simulink model "PMSM_simscape_Model_vs_eq_dq_model"  (R2020b)
settings: Solver=ode23tb  StartTime=0.0  StopTime=0.1  RelTol=1e-4
InitFcn:
  | Ts_sim=20e-06;
  | p=2;
  | phimg=0.125;
  | Zp=2;
  | Rs=2.98;
  | Ld=7e-3;
  | Lq=7e-3;
  | Phimg=0.125;
  | Jm=0.47e-4;
  | Bv=11e-5;
  | TL=0;
  | Vdc=100;
libraries: powerlib x8, powerlib_meascontrol x1
settings Model: ExtModeTrigMode=oneshot  ExtModeArmWhenConnect=off  ExtModeAutoUpdateStatusClock=off  Creator=MathWorks  LastModifiedBy=Karim
settings DataIOCC: ExternalInput=[]  SaveFormat=Array  SignalLoggingSaveFormat=ModelDataLogs  SaveOutput=off  SaveTime=off  ReturnWorkspaceOutputs=off  SignalLoggingName=sigsOut
settings OptimizationCC: BlockReduction=off  BooleanDataType=off  ExpressionDepthLimit=2147483647  InitFltsAndDblsToZero=on  EfficientMapNaN2IntZero=off  LifeSpan=inf
settings DebuggingCC: UnderspecifiedInitializationDetection=Classic  MergeDetectMultiDrivingBlocksExec=none  CheckExecutionContextPreStartOutputMsg=on  CheckExecutionContextRuntimeOutputMsg=on  SignalResolutionControl=TryResolveAllWithWarning  MultiTaskDSMMsg=warning  MultiTaskCondExecSysMsg=none  SigSpecEnsureSampleTimeMsg=none  FcnCallInpInsideContextMsg=warning  StateNameClashWarn=warning  SFUnexpectedBacktrackingDiag=warning  SFNoUnconditionalDefaultTransitionDiag=warning  SFExecutionAtInitializationDiag=none  ArithmeticOperatorsInVariantConditions=warning
settings HardwareCC: ProdBitPerPointer=32  ProdBitPerSizeT=32  ProdBitPerPtrDiffT=32  ProdLargestAtomicFloat=None  ProdIntDivRoundTo=Undefined  ProdEndianess=Unspecified  ProdWordSize=32  ProdHWDeviceType=32-bit Generic  TargetUnknown=on
settings ModelReferenceCC: PropagateSignalLabelsOutOfModel=off
settings SFSimCC: SimUseLocalCustomCode=off  CustomCodeUndefinedFunction=UseInterfaceOnly
settings RTWCC: RTWUseLocalCustomCode=off
settings CodeAppCC: StateflowObjectComments=on
settings GRTTargetCC: TargetLangStandard=C89/C90 (ANSI)  CombineOutputUpdateFcns=off  GRTInterface=on
settings ConfigComp: CovMetricSettings=dw  CovSaveCumulativeToWorkspaceVar=on  CovSaveSingleToWorkspaceVar=on  CovExternalEMLEnable=off  CovSFcnEnable=off
settings SimscapeCC: SimscapeNormalizeSystem=off  SimscapeNominalValues={1, 'bar'; 1, 'cm^3/s'; 1, 'bar*kg/s'; 1, 'kJ/kg'; 1, 'kW'; }

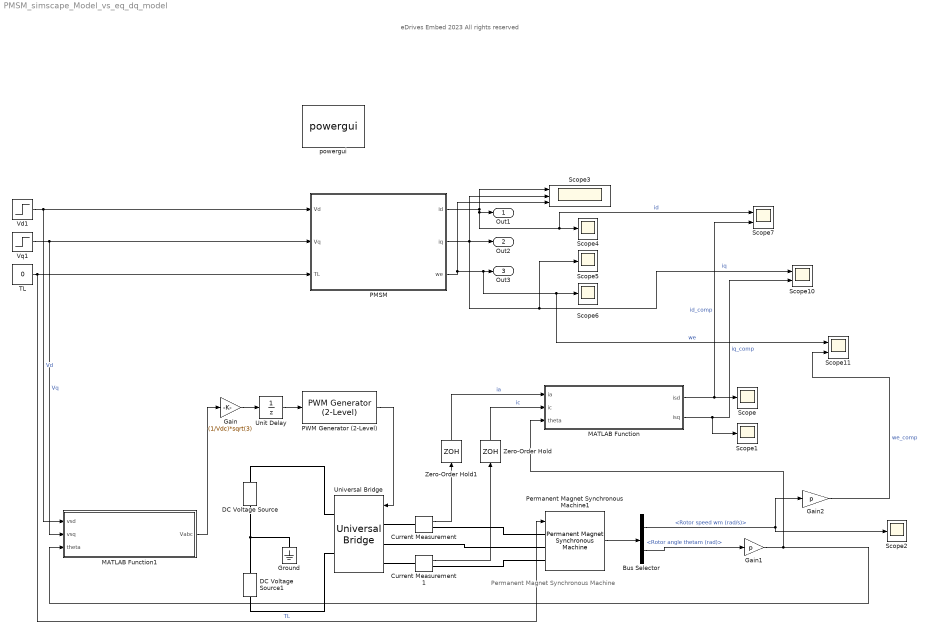
== system PMSM_simscape_Model_vs_eq_dq_model ==
  note: eDrives Embed
      | 2023 All rights reserved
  note: Permanent Magnet Synchronous Machine
  Bus Selector : BusSelector  OutputSignals=Rotor speed wm (rad/s),Rotor angle thetam (rad)
  Current Measurement : powerlib/Measurements/Current Measurement  PhasorSimulation=off  OutputType=Complex  PSBequivalent=0
  Current Measurement1 : powerlib/Measurements/Current Measurement  PhasorSimulation=off  OutputType=Complex  PSBequivalent=0
  DC Voltage Source : powerlib/Electrical Sources/DC Voltage Source  Amplitude=Vdc/2  Measurements=None
  DC Voltage Source1 : powerlib/Electrical Sources/DC Voltage Source  Amplitude=Vdc/2  Measurements=None
  Gain : Gain  Gain=(1/Vdc)*sqrt(3)
  Gain1 : Gain  Gain=p
  Gain2 : Gain  Gain=p
  Ground : powerlib/Elements/Ground  LConnTagsString=a
  MATLAB Function : MATLAB Function  TreatAsAtomicUnit=on
  MATLAB Function1 : MATLAB Function  TreatAsAtomicUnit=on
  PMSM : Subsystem
      mask Display: image('pmsm.png'); % Use "Edit Image" on toolstrip to change.
  PWM Generator (2-Level) : powerlib_meascontrol/Pulse & Signal Generators/PWM Generator (2-Level)  ModulatorType=Three-phase bridge (6 pulses)  ModulatorMode=Unsynchronized  Fc=2e3  Pc=90  nF=27  MinMax="[ -1  1 ]"  SamplingTechnique=Natural  ModulatingSignals=off  m=0.8  Freq=60  Phase=0  Ts=Ts_sim  ShowCarrierOutport=off
  Permanent Magnet Synchronous Machine1 : powerlib/Machines/Permanent Magnet Synchronous Machine  NbPhases=3  FluxDistribution=Sinusoidal  RotorType=Round  MechanicalLoad=Torque Tm  PresetModel=No  ShowDetailedParameters=on  MeasurementBus=off  Resistance=Rs  Inductance=8.5e-3  dqInductances=[8.5e-3,8.5e-3]  La=Ld  MachineConstant=Flux linkage established by magnets (V.s)  Flux=Phimg  VoltageCst=45.345  TorqueCst=0.375  Flat=120  Mechanical=[Jm, Bv p]  PolePairs=4  InitialConditions=[0,0, 0,0]  InitialConditions5ph=[0 0 0 0 0 0]  RefAngle=Aligned with phase A axis (original Park)  IterativeDiscreteModel=Trapezoidal non iterative  TsBlock=-1  TsPowergui=0
  Scope{,1..2,4..6} (6 alike) : Scope
  Scope10 : Scope  NumInputPorts=2
  Scope11 : Scope  NumInputPorts=2
  Scope3 : Scope  NumInputPorts=3
  Scope7 : Scope  NumInputPorts=2
  TL : Constant  Value=0
  Unit Delay : UnitDelay  SampleTime=-1  HasFrameUpgradeWarning=on
  Universal Bridge : powerlib/Power Electronics/Universal Bridge  Arms=3  SnubberResistance=1e5  SnubberCapacitance=inf  Device=IGBT / Diodes  Ron=1e-3  Lon=0  ForwardVoltages="[  0  0  ]"  ForwardVoltage=0  GTOparameters=[ 10e-6 , 20e-6 ]  IGBTparameters=[ 1e-6 , 2e-6 ]  Measurements=None  Measurements_2=None  converterType=Rectifier
  Vd1 : Step  Time=0.001  After=5  SampleTime=0
  Vq1 : Step  Time=0.001  After=20  SampleTime=0
  Zero-Order Hold : ZeroOrderHold  SampleTime=100e-6
  Zero-Order Hold1 : ZeroOrderHold  SampleTime=100e-6
  powergui : powerlib/powergui  Priority=1  SimulationMode=Discrete  SampleTime=Ts_sim  frequency=60  Iterations=50  frequencyindice=0  Pbase=100e6  ErrMax=1e-4  UnitsV=kV  UnitsW=MW  buscounter=0  FunctionMessages=off  echomessages=off  EnableUseOfTLC=off  CurrentSourceSwitches=off  DisableSnubberDevices=off  DisableRonSwitches=off  DisableVfSwitches=off  DisplayEquations=off  AutomaticDiscreteSolvers=off  SolverType=Tustin/Backward Euler (TBE)  Interpol=off  ExternalGateDelay=off  methode=off  Ts=100  x0status=blocks  SPID=on  SwTol=0  HookPort=off  NonlinearTolerance=1e-4  nMaxIteration=100  ContinueOnMaxIteration=off  RestoreLinks=warning  ResistiveCurrentMeasurement=off  Frange=[0:2:500]  Ylog=off  Xlog=on  ShowGrid=off  save=off  variable=ZData  structure=0  ZoomFFT=off  StartTime=0.0  cycles=1  DisplayStyle=1  fundamental=60  FreqAxis=off  MaxFrequency=1000  frequencyindicesteady=1  RmsSteady=1  display=off
  Out1 : Outport
  Out2 : Outport  Port=2
  Out3 : Outport  Port=3
  wires:
  Bus Selector/1 -> Gain2/1, Scope2/1  "<Rotor speed wm (rad/s)>"
  Unit Delay/1 -> PWM Generator (2-Level)/1
  Gain1/1 -> MATLAB Function1/3(theta), MATLAB Function/3(theta)
  MATLAB Function/2(isq) -> Scope10/2, Scope1/1  "iq_comp"
  MATLAB Function/1(isd) -> Scope7/2, Scope/1  "id_comp"
  Gain/1 -> Unit Delay/1
  Zero-Order Hold/1 -> MATLAB Function/2(ic)  "ic"
  MATLAB Function1/1(Vabc) -> Gain/1
  Current Measurement1/1 -> Zero-Order Hold/1
  PWM Generator (2-Level)/1 -> Universal Bridge/1
  Permanent Magnet Synchronous Machine1/1 -> Bus Selector/1
  Zero-Order Hold1/1 -> MATLAB Function/1(ia)  "ia"
  Bus Selector/2 -> Gain1/1  "<Rotor angle thetam (rad)>"
  Current Measurement/1 -> Zero-Order Hold1/1
  Vd1/1 -> MATLAB Function1/1(vsd), PMSM/1(Vd)  "Vd"
  PMSM/1(id) -> Scope7/1, Scope4/1, Out1/1, Scope3/1  "id"
  PMSM/2(iq) -> Scope5/1, Scope10/1, Scope3/2, Out2/1  "iq"
  TL/1 -> PMSM/3(TL), Permanent Magnet Synchronous Machine1/1  "TL"
  PMSM/3(we) -> Scope3/3, Scope11/1, Scope6/1, Out3/1  "we"
  Vq1/1 -> MATLAB Function1/2(vsq), PMSM/2(Vq)  "Vq"
  Gain2/1 -> Scope11/2  "we_comp"
  connections:
  DC Voltage Source/LConn1 -- Ground/LConn1 -- DC Voltage Source1/RConn1
  DC Voltage Source/RConn1 -- Universal Bridge/RConn1
  Permanent Magnet Synchronous Machine1/LConn3 -- Current Measurement1/RConn1
  DC Voltage Source1/LConn1 -- Universal Bridge/RConn2
  Current Measurement/LConn1 -- Universal Bridge/LConn1
  Current Measurement1/LConn1 -- Universal Bridge/LConn3
  Permanent Magnet Synchronous Machine1/LConn1 -- Current Measurement/RConn1
  Permanent Magnet Synchronous Machine1/LConn2 -- Universal Bridge/LConn2

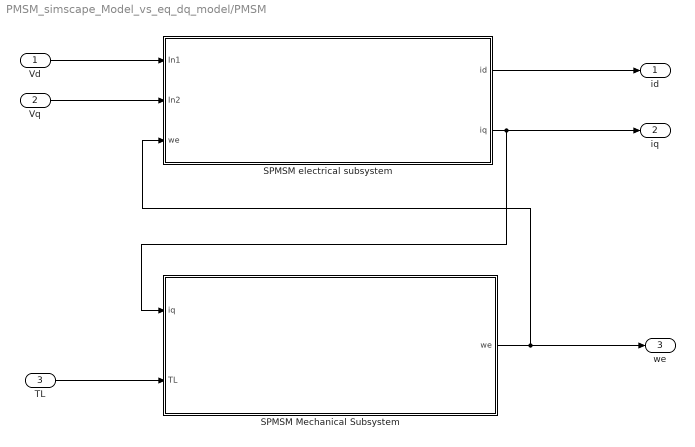
== system PMSM_simscape_Model_vs_eq_dq_model/PMSM ==
  Vd : Inport
  Vq : Inport  Port=2
  TL : Inport  Port=3
  "SPMSM Mechanical Subsystem " : Subsystem
  SPMSM electrical subsystem : Subsystem
  id : Outport
  iq : Outport  Port=2
  we : Outport  Port=3
  wires:
  SPMSM electrical subsystem/2(iq) -> iq/1, "SPMSM Mechanical Subsystem "/1(iq)
  Vd/1 -> SPMSM electrical subsystem/1(In1)
  Vq/1 -> SPMSM electrical subsystem/2(In2)
  SPMSM electrical subsystem/1(id) -> id/1
  "SPMSM Mechanical Subsystem "/1(we) -> we/1, SPMSM electrical subsystem/3(we)
  TL/1 -> "SPMSM Mechanical Subsystem "/2("TL ")

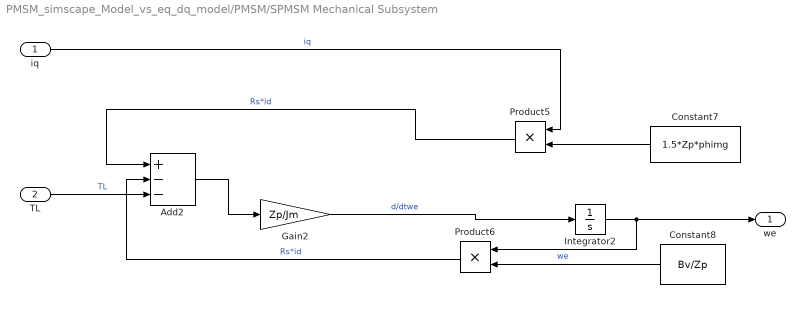
== system PMSM_simscape_Model_vs_eq_dq_model/PMSM/SPMSM Mechanical Subsystem  ==
  iq : Inport
  "TL " : Inport  Port=2
  Add2 : Sum  Inputs=+--
  Constant7 : Constant  Value=1.5*Zp*phimg
  Constant8 : Constant  Value=Bv/Zp
  Gain2 : Gain  Gain=Zp/Jm
  Integrator2 : Integrator
  Product5 : Product
  Product6 : Product
  we : Outport
  wires:
  iq/1 -> Product5/1  "iq"
  Product6/1 -> Add2/2  "Rs*id"
  Integrator2/1 -> we/1, Product6/1  "we"
  "TL "/1 -> Add2/3  "TL"
  Product5/1 -> Add2/1  "Rs*id"
  Constant8/1 -> Product6/2
  Constant7/1 -> Product5/2
  Add2/1 -> Gain2/1
  Gain2/1 -> Integrator2/1  "d/dtwe"

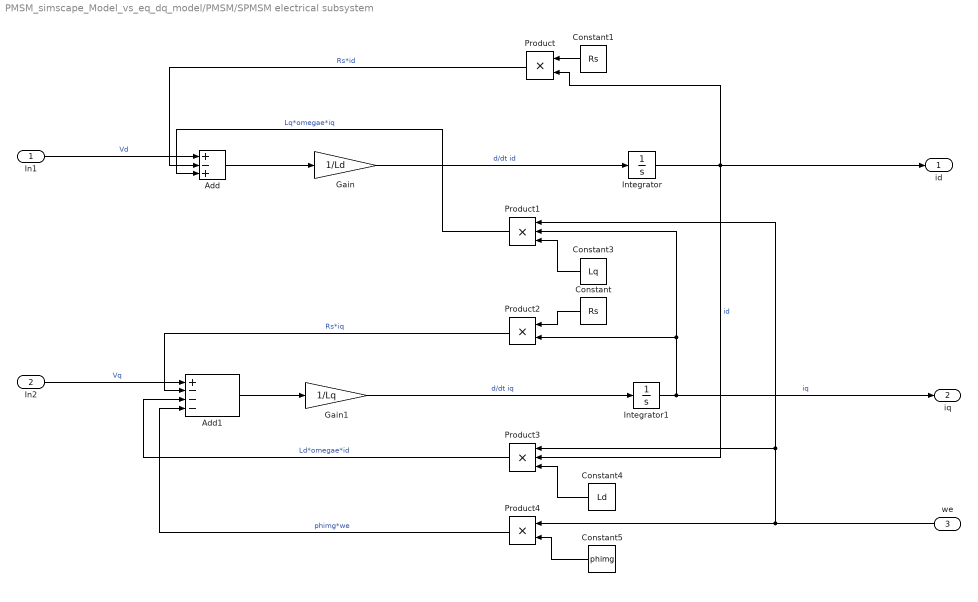
== system PMSM_simscape_Model_vs_eq_dq_model/PMSM/SPMSM electrical subsystem ==
  In1 : Inport
  In2 : Inport  Port=2
  we : Inport  Port=3
  Add : Sum  Inputs=+-+
  Add1 : Sum  Inputs=+---
  Constant : Constant  Value=Rs
  Constant1 : Constant  Value=Rs
  Constant3 : Constant  Value=Lq
  Constant4 : Constant  Value=Ld
  Constant5 : Constant  Value=phimg
  Gain : Gain  Gain=1/Ld
  Gain1 : Gain  Gain=1/Lq
  Integrator : Integrator
  Integrator1 : Integrator
  Product : Product
  Product1 : Product  Inputs=3
  Product2 : Product
  Product3 : Product  Inputs=3
  Product4 : Product
  id : Outport
  iq : Outport  Port=2
  wires:
  Constant5/1 -> Product4/2
  Product1/1 -> Add/3  "Lq*omegae*iq"
  Product/1 -> Add/2  "Rs*id"
  we/1 -> Product4/1, Product3/1, Product1/1
  Constant3/1 -> Product1/3
  Gain/1 -> Integrator/1  "d/dt id"
  Add/1 -> Gain/1
  Constant/1 -> Product2/1
  Gain1/1 -> Integrator1/1  "d/dt iq"
  Constant1/1 -> Product/1
  Product2/1 -> Add1/2  "Rs*iq"
  Integrator/1 -> Product3/2, id/1, Product/2  "id"
  Product4/1 -> Add1/4  "phimg*we"
  Constant4/1 -> Product3/3
  Product3/1 -> Add1/3  "Ld*omegae*id"
  Add1/1 -> Gain1/1
  Integrator1/1 -> iq/1, Product2/2, Product1/2  "iq"
  In1/1 -> Add/1  "Vd"
  In2/1 -> Add1/1  "Vq"

== matlab function PMSM_simscape_Model_vs_eq_dq_model/MATLAB Function1 ==
  data: vsd input; Vabc output; vsq input; theta input
%eDrives Embed


function Vabc= Inv_Park_Clarke_Voltage(vsd,vsq,theta)



% initial condition for theta

if isempty(theta)
theta=0;
end



T=[1 0;-1/2 sqrt(3)/2;-1/2 -sqrt(3)/2]...
*[cos(theta) -sin(theta);sin(theta) cos(theta)];

Vabc=T*[vsd;vsq];

== matlab function PMSM_simscape_Model_vs_eq_dq_model/MATLAB Function ==
  data: ia input; isd output; ic input; theta input; isq output
%% eDrives Embed
function [isd,isq]= Park_Clarke_Current(ia,ic,theta)


%initial condition fot theta

if isempty(theta)       
theta=0;
end

%Park-Clarke transform

isd = cos(theta)*ia+sin(theta)*(-sqrt(3)/3*ia-2*sqrt(3)/3*ic);
isq = -sin(theta)*ia+cos(theta)*(-sqrt(3)/3*ia-2*sqrt(3)/3*ic);
